simulink model "testFrame_rf_sbstm_disable_integrator_on_start_up"  (R2022b)
settings: Solver=FixedStepDiscrete  StartTime=0.0  StopTime=30  FixedStep=0.01  RelTol=1e-3
libraries: simulink x1
settings Model: PacingRate=0.100000  Creator=unix  LastModifiedBy=unix
settings SolverCC: AlgebraicLoopSolver=TrustRegion
settings DebuggingCC: IntegerOverflowMsg=error  ParameterUnderflowMsg=error  UnconnectedInputMsg=warning  UnconnectedOutputMsg=warning  UnconnectedLineMsg=warning  SFMachineParentedDataDiag=warning  IntegerSaturationMsg=error
settings ModelReferenceCC: EnableRefExpFcnMdlSchedulingChecks=on
settings RTWCC: DLArmComputeVersion=19.05

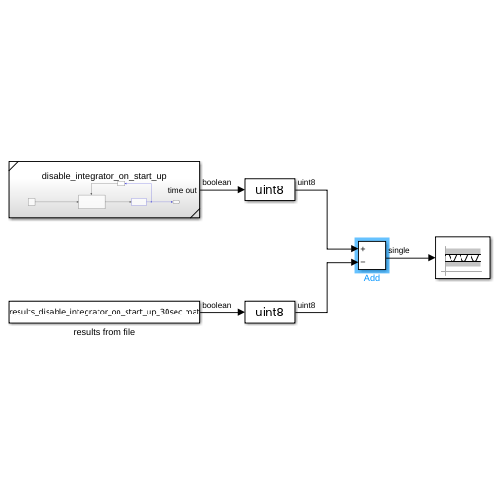
[thumbnail: Simulink's stored preview of the top-level diagram]
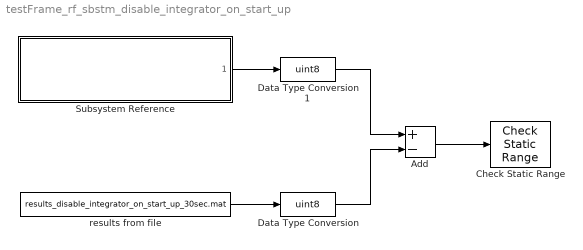
== system testFrame_rf_sbstm_disable_integrator_on_start_up ==
  Add : Sum  Inputs=+-  OutDataTypeStr=single
  Check Static Range : simulink/Model Verification/Check  Static Range  Description=-0.1 <= u <= 0  max=0  max_included=on  min=-0.1  min_included=on  enabled=on  stopWhenAssertionFail=on  export=off  icon=graphic
  Data Type Conversion : DataTypeConversion  OutDataTypeStr=uint8  SaturateOnIntegerOverflow=off  RndMeth=Floor
  Data Type Conversion1 : DataTypeConversion  OutDataTypeStr=uint8  SaturateOnIntegerOverflow=off  RndMeth=Floor
  Subsystem Reference : Subsystem  ReferencedSubsystem=disable_integrator_on_start_up
  results from file : FromFile  FileName=results_disable_integrator_on_start_up_30sec.mat
  wires:
  Subsystem Reference/1 -> Data Type Conversion1/1
  results from file/1 -> Data Type Conversion/1
  Data Type Conversion1/1 -> Add/1
  Data Type Conversion/1 -> Add/2
  Add/1 -> Check Static Range/1
